simulink model "trial"  (R2020a)
settings: Solver=VariableStepAuto  StartTime=0.0  StopTime=600.0  RelTol=1e-3
libraries: cstblocks x3
settings Model: Creator=vivek  LastModifiedBy=vivek

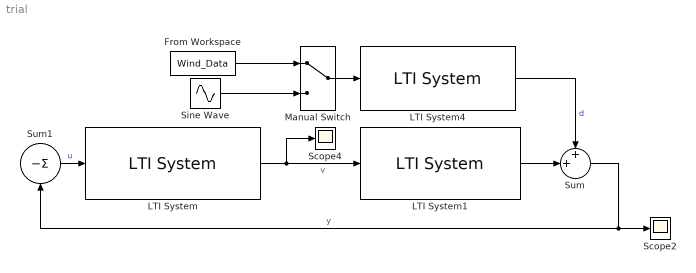
== system trial ==
  From Workspace : FromWorkspace  VariableName=Wind_Data
  LTI System : cstblocks/LTI System  sys=ktf21  IC=[]
  LTI System1 : cstblocks/LTI System  sys=sg21w  IC=[]
  LTI System4 : cstblocks/LTI System  sys=Gd21  IC=[]
  Manual Switch : ManualSwitch
  Scope2 : Scope
  Scope4 : Scope
  Sine Wave : Sin  SampleTime=0
  Sum : Sum  Inputs=++|
  Sum1 : Sum  Inputs=|-
  wires:
  LTI System/1 -> Scope4/1, LTI System1/1  "v"
  Sum/1 -> Sum1/1, Scope2/1  "y"
  LTI System4/1 -> Sum/1  "d"
  LTI System1/1 -> Sum/2
  Sum1/1 -> LTI System/1  "u"
  Manual Switch/1 -> LTI System4/1
  From Workspace/1 -> Manual Switch/1
  Sine Wave/1 -> Manual Switch/2
